simulink model "Example_4_16_model"  (R2017a)
settings: Solver=ode4  StartTime=0.0  StopTime=10  FixedStep=0.01  RelTol=1e-3
values from neighbouring files (symbols this model uses):
  A = [a -b;b a]    [Example_4_16.m]
  B = [0 1]'    [Example_4_16.m]
  C = [1 0]    [Example_4_16.m]
  L = acker(A',C',lambda_obs_des)'    [Example_4_16.m]
  x0 = [-1.5 0.25]'    [Example_4_16.m]
  xhat0 = 5*x0    [Example_4_16.m]
settings Model: Creator=roga  LastModifiedBy=Roberto
settings DataIOCC: LimitDataPoints=on  SaveFormat=Array
settings OptimizationCC: LifeSpan=inf
settings DebuggingCC: UnderspecifiedInitializationDetection=Classic  MergeDetectMultiDrivingBlocksExec=none  SolverPrmCheckMsg=warning  StateNameClashWarn=warning  SFUnexpectedBacktrackingDiag=warning  SFNoUnconditionalDefaultTransitionDiag=warning  SFExecutionAtInitializationDiag=none
settings HardwareCC: ProdBitPerPointer=32  ProdBitPerSizeT=32  ProdBitPerPtrDiffT=32  ProdLargestAtomicFloat=None  ProdIntDivRoundTo=Undefined  ProdEndianess=Unspecified  ProdWordSize=32  ProdHWDeviceType=32-bit Generic
settings ModelReferenceCC: PropagateSignalLabelsOutOfModel=off
settings GRTTargetCC: TargetLangStandard=C89/C90 (ANSI)  GeneratePreprocessorConditionals=Disable all
settings ConfigComp: CovMetricSettings=dw  CovHtmlReporting=on  CovSaveCumulativeToWorkspaceVar=on  CovSaveSingleToWorkspaceVar=on  CovExternalEMLEnable=off

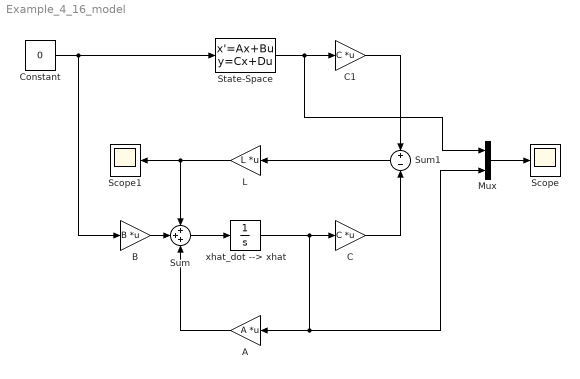
== system Example_4_16_model ==
  A : Gain  Gain=A  Multiplication=Matrix(K*u) (u vector)
  B : Gain  Gain=B  Multiplication=Matrix(K*u) (u vector)
  C : Gain  Gain=C  Multiplication=Matrix(K*u) (u vector)
  C1 : Gain  Gain=C  Multiplication=Matrix(K*u) (u vector)
  Constant : Constant  Value=0
  L : Gain  Gain=L  Multiplication=Matrix(K*u) (u vector)
  Mux : Mux  Inputs=2
  Scope : Scope
  Scope1 : Scope
  State-Space : StateSpace  A=A  B=B  C=eye(2)  D=zeros(2,1)  X0=x0
  Sum : Sum  Inputs=+++
  Sum1 : Sum  Inputs=+-
  xhat_dot --> xhat : Integrator  InitialCondition=xhat0
  wires:
  Constant/1 -> B/1, State-Space/1
  Mux/1 -> Scope/1
  Sum/1 -> xhat_dot --> xhat/1
  B/1 -> Sum/2
  A/1 -> Sum/3
  L/1 -> Scope1/1, Sum/1
  Sum1/1 -> L/1
  C/1 -> Sum1/2
  C1/1 -> Sum1/1
  State-Space/1 -> Mux/1, C1/1
  xhat_dot --> xhat/1 -> C/1, A/1, Mux/2
